simulink model "momentum_observer"  (R2025a)
settings: Solver=ode15s  StartTime=0.0  StopTime=10.0  MaxStep=0.01  RelTol=1e-4  AbsTol=1e-7
libraries: robotmaniplib x3
settings Model: Creator=visc1  LastModifiedBy=visc1

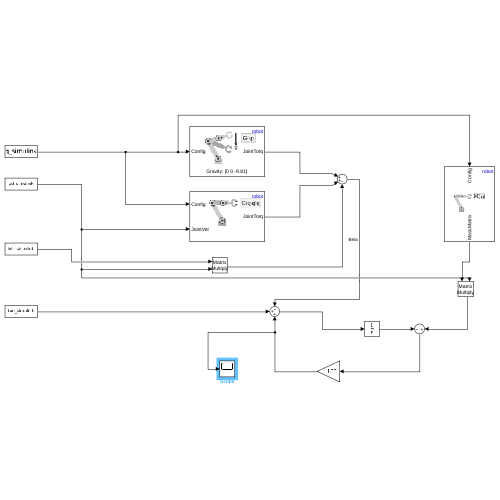
[thumbnail: Simulink's stored preview of the top-level diagram]
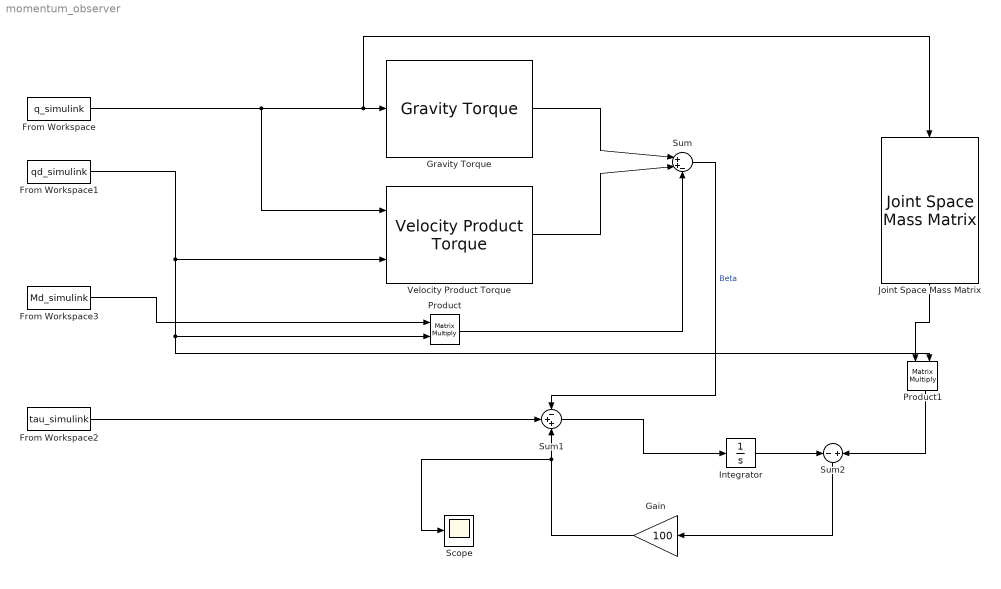
== system momentum_observer ==
  From Workspace : FromWorkspace  VariableName=q_simulink
  From Workspace1 : FromWorkspace  VariableName=qd_simulink
  From Workspace2 : FromWorkspace  VariableName=tau_simulink
  From Workspace3 : FromWorkspace  VariableName=Md_simulink
  Gain : Gain  Gain=100
  Gravity Torque : robotmaniplib/Gravity Torque  RigidBodyTree=robot  SimulateUsing=Interpreted execution
  Integrator : Integrator
  Joint Space Mass Matrix : robotmaniplib/Joint Space Mass Matrix  RigidBodyTree=robot  SimulateUsing=Interpreted execution
  Product : Product  Multiplication=Matrix(*)
  Product1 : Product  Multiplication=Matrix(*)
  Scope : Scope
      settings: ActiveDisplayYMinimum=-0.14934775789101551  ActiveDisplayYMaximum=0.035190105310328526
  Sum : Sum  Inputs=|++-
  Sum1 : Sum  Inputs=-++
  Sum2 : Sum  Inputs=-|+
  Velocity Product Torque : robotmaniplib/Velocity Product Torque  RigidBodyTree=robot  SimulateUsing=Interpreted execution
  wires:
  From Workspace/1 -> Gravity Torque/1, Joint Space Mass Matrix/1, Velocity Product Torque/1
  Gravity Torque/1 -> Sum/1
  Velocity Product Torque/1 -> Sum/2
  From Workspace3/1 -> Product/1
  Product/1 -> Sum/3
  From Workspace2/1 -> Sum1/2
  Sum/1 -> Sum1/1  "Beta"
  Sum1/1 -> Integrator/1
  Integrator/1 -> Sum2/1
  Joint Space Mass Matrix/1 -> Product1/1
  From Workspace1/1 -> Product1/2, Product/2, Velocity Product Torque/2
  Product1/1 -> Sum2/2
  Sum2/1 -> Gain/1
  Gain/1 -> Scope/1, Sum1/3
